simulink model "Part1"  (R2023b)
settings: Solver=VariableStepAuto  StartTime=0.0  StopTime=0.021  RelTol=1e-3
undefined symbols (not defined in the file): NBits
libraries: fl_lib x29, nesl_utility x8, ee_lib x3, msbAdcArchitectures x1
settings Model: Creator=firas  LastModifiedBy=firas

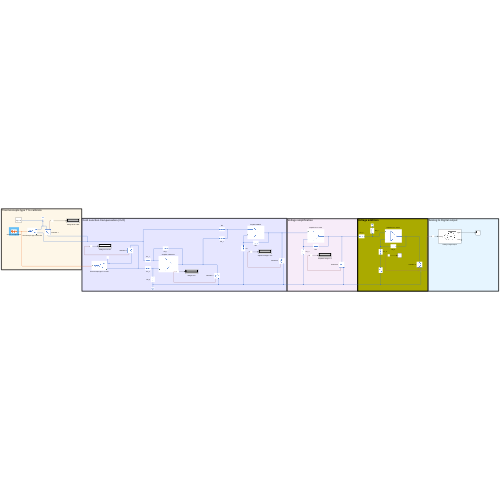
[thumbnail: Simulink's stored preview of the top-level diagram]
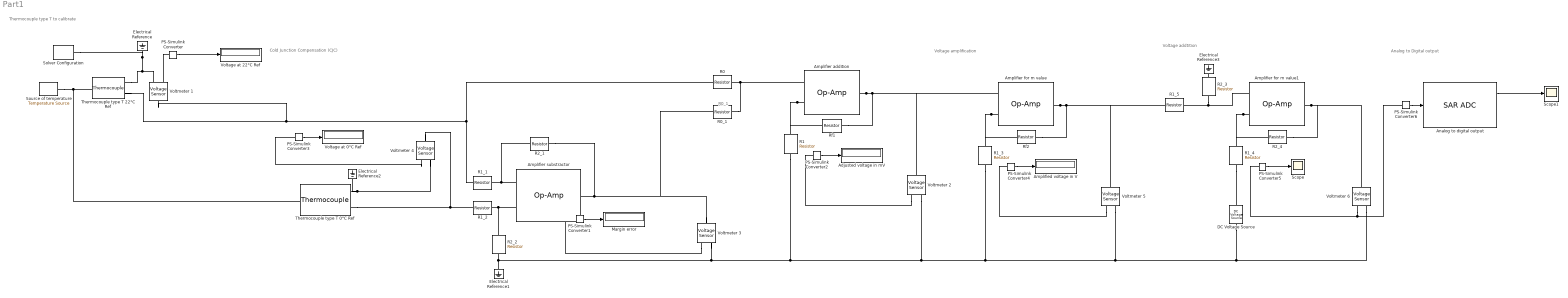
== system Part1 ==
  note: Voltage amplification
  note: Thermocouple type T to calibrate
  note: Cold Junction Compensation (CJC)
  note: R0_1
  note: Voltage addtition
  note: Analog to Digital output
  Adjusted voltage in mV : Display
      settings: Decimation=1000
  Amplified voltage in V : Display
      settings: Decimation=1000
  Amplifier addition : fl_lib/Electrical/Electrical Elements/Op-Amp  outI_specify=off  outI_priority=None  outI=0 A  outI_nominal_specify=off  outI_nominal_unit=A  outI_nominal_value=1
  Amplifier for m value : fl_lib/Electrical/Electrical Elements/Op-Amp  outI_specify=off  outI_priority=None  outI=0 A  outI_nominal_specify=off  outI_nominal_unit=A  outI_nominal_value=1
  Amplifier for m value1 : fl_lib/Electrical/Electrical Elements/Op-Amp  outI_specify=off  outI_priority=None  outI=0 A  outI_nominal_specify=off  outI_nominal_unit=A  outI_nominal_value=1
  Amplifier substractor : fl_lib/Electrical/Electrical Elements/Op-Amp  outI_specify=off  outI_priority=None  outI=0 A  outI_nominal_specify=off  outI_nominal_unit=A  outI_nominal_value=1
  Analog to digital output : msbAdcArchitectures/SAR ADC  DACVoltages=[-5:5]  DACINLVoltages=tanh([-5:5])  NBits=8  InputRange=[1.012 6.012]  ExtStartClk=off  StartFreq=10e1  StartClkJitter=0  SARFreq=2e7  MatchScale=off  OutputPolarity=Auto  OutDataType=fixdt(0,NBits)  EnableLinearityImpairments=off  OffsetError=1  OffsetErrorUnit=LSB  GainError=2  GainErrorUnit=LSB
  DC Voltage Source : ee_lib/Additional Components/SPICE Sources/DC Voltage Source  DC=4.0510453946129 V
  Electrical Reference{,1..3} (4 alike) : fl_lib/Electrical/Electrical Elements/Electrical Reference
  Margin error : Display
      settings: Decimation=1000
  PS-Simulink Converter{,1..6} (7 alike) : nesl_utility/PS-Simulink Converter  PhysicalDomain=network_engine_domain  SubClassName=ps_output  LeftPortType=input  RightPortType=output  PseudoPeriodic=off  Frequencies=[]  VectorFormat=inherit  Unit=inherit  AffineConversion=off
  R0 : fl_lib/Electrical/Electrical Elements/Resistor  R=10 Ohm  i_specify=off  i_priority=None  i=0 A  i_nominal_specify=off  i_nominal_unit=A  i_nominal_value=1  v_specify=off  v_priority=None  v=0 V  v_nominal_specify=off  v_nominal_unit=V  v_nominal_value=1
  R0_1 : fl_lib/Electrical/Electrical Elements/Resistor  R=10 Ohm  i_specify=off  i_priority=None  i=0 A  i_nominal_specify=off  i_nominal_unit=A  i_nominal_value=1  v_specify=off  v_priority=None  v=0 V  v_nominal_specify=off  v_nominal_unit=V  v_nominal_value=1
  R1 : fl_lib/Electrical/Electrical Elements/Resistor  R=10 Ohm  i_specify=off  i_priority=None  i=0 A  i_nominal_specify=off  i_nominal_unit=A  i_nominal_value=1  v_specify=off  v_priority=None  v=0 V  v_nominal_specify=off  v_nominal_unit=V  v_nominal_value=1
  R1_{1..5} (5 alike) : fl_lib/Electrical/Electrical Elements/Resistor  R=10 Ohm  i_specify=off  i_priority=None  i=0 A  i_nominal_specify=off  i_nominal_unit=A  i_nominal_value=1  v_specify=off  v_priority=None  v=0 V  v_nominal_specify=off  v_nominal_unit=V  v_nominal_value=1
  R2_{1..4} (4 alike) : fl_lib/Electrical/Electrical Elements/Resistor  R=10 Ohm  i_specify=off  i_priority=None  i=0 A  i_nominal_specify=off  i_nominal_unit=A  i_nominal_value=1  v_specify=off  v_priority=None  v=0 V  v_nominal_specify=off  v_nominal_unit=V  v_nominal_value=1
  Rf1 : fl_lib/Electrical/Electrical Elements/Resistor  R=10 Ohm  i_specify=off  i_priority=None  i=0 A  i_nominal_specify=off  i_nominal_unit=A  i_nominal_value=1  v_specify=off  v_priority=None  v=0 V  v_nominal_specify=off  v_nominal_unit=V  v_nominal_value=1
  Rf2 : fl_lib/Electrical/Electrical Elements/Resistor  R=7534.3755886231 Ohm  i_specify=off  i_priority=None  i=0 A  i_nominal_specify=off  i_nominal_unit=A  i_nominal_value=1  v_specify=off  v_priority=None  v=0 V  v_nominal_specify=off  v_nominal_unit=V  v_nominal_value=1
  Scope : Scope
  Scope1 : Scope
  Solver Configuration : nesl_utility/Solver Configuration  PhysicalDomain=network_engine_domain  SubClassName=solver  LeftPortType=input  RightPortType=generic  Tones=[]  Harmonics=[]  SimulateNoise=off  Profile=off  UseLocalSampling=off  EnableSwitchedLinearOptims=on  FrequencyDomain=off  UseCCode=off  RelTol=0.001  AbsTol=0.001  MinStep=1e-09  ToWorkspace=off  RevertToSquareIcSolve=off  NumHomotopyIterations=100  PhasorMode=off  PhasorModeNumHarmonics=1  ConsistencySolver=NEWTON_XTOL_AFTER_FTOL  IndexReductionMethod=DerivativeReplacement  DoDC=off  ResidualTolerance=1e-09  ConsistencyTolSource=GLOBAL  ConsistencyAbsTol=0.001  ConsistencyRelTol=0.001  ConsistencyTolFactor=0.001  UseLocalSolver=off  LocalSolverChoice=NE_BACKWARD_EULER_ADVANCER  ResolveIndetEquations=on  FunctionEvalNumThread=1  LocalSolverSampleTime=0.001  DoFixedCost=off  MaxNonlinIter=3  MaxModeIter=2  ComputeImpulses=off  ImpulseIterations=2  LinearAlgebra=auto  LinearAlgebraNumThread=0  EquationFormulation=NE_TIME_EF  DelaysMemoryBudget=1024  AutomaticFiltering=on  FilteringTimeConstant=0.001  PartitionStorageMethod=AS_NEEDED  PartitionMemoryBudget=1024  PartitionMethod=ROBUST  MultibodyUseLocalSolver=off  MultibodyLocalSolverChoice=ODE1  MultibodyLocalSolverSampleTime=0.001
  Source of temperature : fl_lib/Thermal/Thermal Sources/Temperature Source  temperature=160 degC
  Thermocouple type T 0°C Ref : ee_lib/Sensors & Transducers/Thermocouple  thermocouple_type=1  Cvec=[0.000000000000E+00, 0.387481063640E-01, 0.332922278800E-04, 0.206182434040E-06, -0.218822568460E-08, 0.109968809280E-10, -0.308157587720E-13, 0.454791352900E-16, -0.275129016730E-19]  Avec=[0, 0, 0]  T0=0 degC  tc=1 s  K_d=1e-3 W/K  init_temp=150 degC
      settings: InternalSimscapePortConfiguration="{\"Bottom\":[],\"Left\":[{\"id\":\"p\",\"label\":\"+\",\"type\":\"foundation.electrical.electrical\"},{\"id\":\"n\",\"label\":\"-\",\"type\":\"foundation.electrical.electrical\"}],\"Right\":[{\"id\":\"A\",\"label\":\"A\",\"type\":\"foundation.thermal.thermal\"}],\"Top\":[]}"
  Thermocouple type T 22°C Ref : ee_lib/Sensors & Transducers/Thermocouple  thermocouple_type=1  Cvec=[0.000000000000E+00, 0.387481063640E-01, 0.332922278800E-04, 0.206182434040E-06, -0.218822568460E-08, 0.109968809280E-10, -0.308157587720E-13, 0.454791352900E-16, -0.275129016730E-19]  Avec=[0, 0, 0]  T0=22 degC  tc=1 s  K_d=1e-3 W/K  init_temp=150 degC
      settings: InternalSimscapePortConfiguration="{\"Bottom\":[],\"Left\":[{\"id\":\"p\",\"label\":\"+\",\"type\":\"foundation.electrical.electrical\"},{\"id\":\"n\",\"label\":\"-\",\"type\":\"foundation.electrical.electrical\"}],\"Right\":[{\"id\":\"A\",\"label\":\"A\",\"type\":\"foundation.thermal.thermal\"}],\"Top\":[]}"
  Voltage at 0°C Ref : Display
      settings: Decimation=1000
  Voltage at 22°C Ref : Display
      settings: Decimation=1000
  Voltmeter {1..6} (6 alike) : fl_lib/Electrical/Electrical Sensors/Voltage Sensor
  wires:
  PS-Simulink Converter1/1 -> Margin error/1
  PS-Simulink Converter/1 -> Voltage at 22°C Ref/1
  PS-Simulink Converter2/1 -> Adjusted voltage in mV/1
  PS-Simulink Converter3/1 -> Voltage at 0°C Ref/1
  PS-Simulink Converter4/1 -> Amplified voltage in V/1
  PS-Simulink Converter5/1 -> Scope/1
  PS-Simulink Converter6/1 -> Analog to digital output/1
  Analog to digital output/1 -> Scope1/1
  connections:
  Source of temperature/LConn1 -- Thermocouple type T 0°C Ref/RConn1 -- Thermocouple type T 22°C Ref/RConn1
  Thermocouple type T 22°C Ref/LConn2 -- Voltmeter 1/RConn2 -- Electrical Reference/LConn1 -- Solver Configuration/RConn1
  PS-Simulink Converter/LConn1 -- Voltmeter 1/RConn1
  Thermocouple type T 22°C Ref/LConn1 -- R1_1/RConn1 -- R0/RConn1 -- Voltmeter 1/LConn1
  Thermocouple type T 0°C Ref/LConn1 -- Voltmeter 4/LConn1 -- R1_2/RConn1
  Amplifier substractor/LConn2 -- R2_1/LConn1 -- R1_1/LConn1
  Amplifier substractor/LConn1 -- R2_2/LConn1 -- R1_2/LConn1
  Voltmeter 6/RConn2 -- DC Voltage Source/RConn1 -- Electrical Reference1/LConn1 -- R2_2/RConn1 -- Voltmeter 3/RConn2 -- R1/LConn1 -- Voltmeter 2/RConn2 -- R1_3/LConn1 -- Voltmeter 5/RConn2
  R2_1/RConn1 -- R0_1/RConn1 -- Voltmeter 3/LConn1 -- Amplifier substractor/RConn1
  Voltmeter 3/RConn1 -- PS-Simulink Converter1/LConn1
  Thermocouple type T 0°C Ref/LConn2 -- Electrical Reference2/LConn1 -- Voltmeter 4/RConn2
  Amplifier addition/RConn1 -- Voltmeter 2/LConn1 -- Amplifier for m value/LConn1 -- Rf1/RConn1
  Amplifier addition/LConn1 -- R0_1/LConn1 -- R0/LConn1
  Amplifier addition/LConn2 -- Rf1/LConn1 -- R1/RConn1
  Voltmeter 2/RConn1 -- PS-Simulink Converter2/LConn1
  Voltmeter 4/RConn1 -- PS-Simulink Converter3/LConn1
  Amplifier for m value/LConn2 -- Rf2/LConn1 -- R1_3/RConn1
  Amplifier for m value/RConn1 -- R1_5/RConn1 -- Voltmeter 5/LConn1 -- Rf2/RConn1
  Voltmeter 5/RConn1 -- PS-Simulink Converter4/LConn1
  Amplifier for m value1/LConn2 -- R2_4/LConn1 -- R1_4/RConn1
  Amplifier for m value1/RConn1 -- R2_4/RConn1 -- Voltmeter 6/LConn1
  Voltmeter 6/RConn1 -- PS-Simulink Converter6/LConn1 -- PS-Simulink Converter5/LConn1
  Amplifier for m value1/LConn1 -- R1_5/LConn1 -- R2_3/LConn1
  Electrical Reference3/LConn1 -- R2_3/RConn1
  R1_4/LConn1 -- DC Voltage Source/LConn1
